simulink model "gm_sampleModel1476_sub"  (R2023a)
settings: Solver=VariableStepAuto  StartTime=0.0  StopTime=10.0  RelTol=1e-3
libraries: simulink x1
settings Model: Creator=user1  LastModifiedBy=user1
settings OptimizationCC: BlockReduction=off  ConditionallyExecuteInputs=off
settings DebuggingCC: InheritedTsInSrcMsg=none

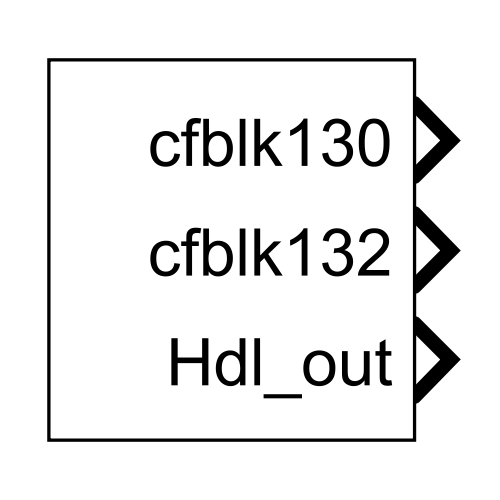
[thumbnail: Simulink's stored preview of the top-level diagram]
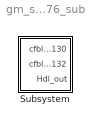
== system gm_sampleModel1476_sub ==
  Subsystem : Subsystem

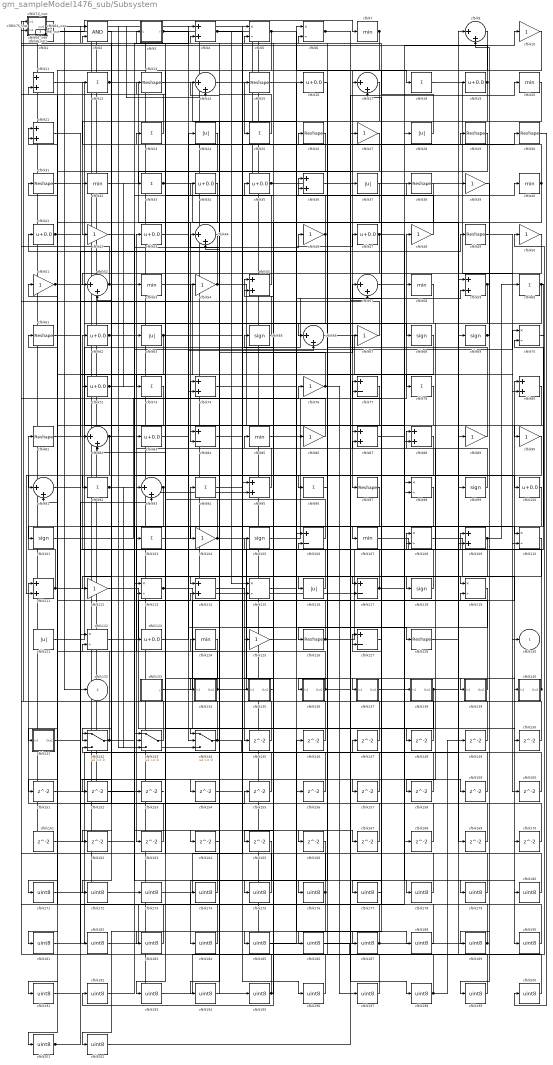
== system gm_sampleModel1476_sub/Subsystem ==
  cfblk1 : simulink/Logic and Bit Operations/Extract Bits  bitsToExtract=Upper half  numBits=8  bitIdxRange=[0 7]  outScalingMode=Preserve fixed-point scaling
      settings: LibrarySourceBlock=|
      | hdlsllib/Logic and Bit
      | Operations/Extract Bits
  cfblk{10,27,39,42,46,48,50..51,54,67,76,86,89..90,104,112,125} (17 alike) : Gain  OutDataTypeStr=uint8
  cfblk{16,19,34..35,41,43,47,62,72,83,100,123} (12 alike) : Bias  Bias=0.0  SaturateOnIntegerOverflow=off
  cfblk{65,68..69,99,101,105,118} (7 alike) : Signum
  cfblk102_inst : Subsystem
  cfblk{12,18,23,25,33,60,73,78,92,94,96,103} (12 alike) : Sum  Inputs=+  OutDataTypeStr=uint8
  cfblk{77,84,106,117,127} (5 alike) : Sum  Inputs=+-  OutDataTypeStr=uint8
  cfblk{7,20,32,40,53,58,85,107,124} (9 alike) : MinMax  OutDataTypeStr=uint8
  cfblk{5..6,70,98,108,110,113,115,119,122} (10 alike) : Product  Inputs=*/  OutDataTypeStr=uint8  RndMeth=Zero  SaturateOnIntegerOverflow=on
  cfblk{4,11,21,36,55,59,74,80,87..88,95,109,111,114} (14 alike) : Sum  OutDataTypeStr=uint8
  cfblk{24,28,37,63,116,121} (6 alike) : Abs  OutDataTypeStr=uint8  SaturateOnIntegerOverflow=off
  cfblk120_inst : Subsystem
  cfblk{13,15,26,29..31,38,49,61,81,97,126,128} (13 alike) : Reshape
  cfblk133 : Subsystem  mask(Counter Free-Running){NumBits=double(16), tsamp=double(-1)}
      mask prompts: NumBits "Simulink:masks:NumberOfBits_MP"; tsamp "Simulink:masks:SampleTime_MP"
      mask help: Simulink:masks:CounterFreeRunning_MD
  cfblk134 : Subsystem
  cfblk135 : Subsystem
  cfblk136 : Subsystem
  cfblk137 : Subsystem
  cfblk138 : Subsystem
  cfblk139 : Subsystem
  cfblk{9,14,17,44,52,57,66,82,91,93} (10 alike) : Sum  Inputs=|++  OutDataTypeStr=uint8
  cfblk140 : Subsystem
  cfblk141 : Subsystem
  cfblk142 : Switch  OutDataTypeStr=uint8  SaturateOnIntegerOverflow=off  InputSameDT=off
  cfblk143 : Switch  OutDataTypeStr=uint8  SaturateOnIntegerOverflow=off  InputSameDT=off
  cfblk144 : Switch  OutDataTypeStr=uint8  SaturateOnIntegerOverflow=off  InputSameDT=off
  cfblk{145..170} (26 alike) : Delay  SampleTime=1
  cfblk{171..202} (32 alike) : DataTypeConversion  OutDataTypeStr=uint8  SaturateOnIntegerOverflow=off  RndMeth=Floor
  cfblk2 : Logic  AllPortsSameDT=off  OutDataTypeStr=boolean
  cfblk3 : Subsystem  mask(Detect Rise Positive){vinit=double(0), InputProcessing=Elements as channels (sample based), OutDataTypeStr=uint8}
      mask prompts: vinit "Simulink:masks:InitialCondition_MP"; InputProcessing "Simulink:masks:InputProcessing_MP"; OutDataTypeStr "Simulink:masks:OutputDataType_MP"
      mask help: Simulink:masks:DetectRisePositive_MD
      mask init:
      | InputProcessing = 'Elements as channels (sample based)';
      | OutDataTypeStr = 'uint8';
      | vinit = double(0);
      mask TypeOptions InputProcessing: Simulink:masks:ColumnsAsChannelsFrameBased | Simulink:masks:ElementsAsChannelsSampleBased
      mask TypeOptions OutDataTypeStr: Simulink:masks:uint8 | Simulink:masks:boolean
      mask Display: fprintf('U > 0\n&  NOT\nU/z > 0')
  cfblk45_inst : Subsystem
  cfblk56_inst : Subsystem
  cfblk64_inst : Subsystem
  cfblk71_inst : Subsystem
  cfblk75_inst : Subsystem
  cfblk8_inst : Subsystem
  cfblk130 : Outport  OutDataTypeStr=uint8  SampleTime=1  VectorParamsAs1DForOutWhenUnconnected=off
  cfblk132 : Outport  Port=2  OutDataTypeStr=uint8  SampleTime=1  VectorParamsAs1DForOutWhenUnconnected=off
  Hdl_out : Outport  Port=3  OutDataTypeStr=uint8  SampleTime=1
  wires:
  cfblk1/1 -> cfblk7/1
  cfblk10/1 -> cfblk97/1
  cfblk100/1 -> cfblk163/1
  cfblk101/1 -> cfblk76/1
  cfblk102_inst/1(out1) -> cfblk173/1
  cfblk103/1 -> cfblk94/1
  cfblk104/1 -> cfblk82/2, cfblk119/1, cfblk137/1(In1)
  cfblk105/1 -> cfblk48/1
  cfblk106/1 -> cfblk8_inst/1(in1)
  cfblk107/1 -> cfblk70/2
  cfblk108/1 -> cfblk190/1
  cfblk109/1 -> cfblk143/2, cfblk60/1
  cfblk11/1 -> cfblk87/1
  cfblk110/1 -> cfblk114/1
  cfblk111/1 -> cfblk81/1, cfblk118/1
  cfblk112/1 -> cfblk170/1
  cfblk113/1 -> cfblk30/1, cfblk150/1
  cfblk114/1 -> cfblk145/1
  cfblk115/1 -> cfblk16/1
  cfblk116/1 -> cfblk43/1
  cfblk117/1 -> cfblk105/1, cfblk10/1
  cfblk118/1 -> cfblk62/1
  cfblk119/1 -> cfblk126/1
  cfblk12/1 -> cfblk84/2, cfblk142/2
  cfblk120_inst/1(out1) -> cfblk95/2
  cfblk121/1 -> cfblk59/2
  cfblk122/1 -> cfblk114/2
  cfblk123/1 -> cfblk24/1
  cfblk124/1 -> cfblk193/1
  cfblk125/1 -> cfblk58/1
  cfblk126/1 -> cfblk109/1, cfblk51/1
  cfblk127/1 -> cfblk187/1
  cfblk128/1 -> cfblk89/1
  cfblk13/1 -> cfblk106/1
  cfblk133/1(y) -> cfblk80/1
  cfblk134/1(Out1) -> cfblk9/1, cfblk61/1
  cfblk135/1(Out1) -> cfblk55/1
  cfblk136/1(Out1) -> cfblk93/1, cfblk119/2, cfblk20/1
  cfblk137/1(Out1) -> cfblk98/2
  cfblk138/1(Out1) -> cfblk69/1, cfblk153/1
  cfblk139/1(Out1) -> cfblk44/1
  cfblk14/1 -> cfblk25/1
  cfblk140/1(Out1) -> cfblk88/1, cfblk83/1
  cfblk141/1(Out1) -> cfblk154/1
  cfblk142/1 -> cfblk123/1, cfblk46/1, cfblk164/1, cfblk122/2
  cfblk143/1 -> cfblk72/1
  cfblk144/1 -> cfblk147/1, cfblk113/2
  cfblk145/1 -> cfblk14/1
  cfblk146/1 -> cfblk120_inst/2(in2)
  cfblk147/1 -> cfblk8_inst/2(in2)
  cfblk148/1 -> cfblk87/2
  cfblk149/1 -> cfblk11/2
  cfblk15/1 -> cfblk156/1
  cfblk150/1 -> cfblk64_inst/2(in2)
  cfblk151/1 -> cfblk59/1
  cfblk152/1 -> cfblk74/1
  cfblk153/1 -> cfblk1/1
  cfblk154/1 -> cfblk115/2
  cfblk155/1 -> cfblk142/3
  cfblk156/1 -> cfblk95/1
  cfblk157/1 -> cfblk44/2
  cfblk158/1 -> cfblk6/2
  cfblk159/1 -> cfblk2/2
  cfblk16/1 -> cfblk96/1
  cfblk160/1 -> cfblk106/2
  cfblk161/1 -> cfblk143/1
  cfblk162/1 -> cfblk70/1
  cfblk163/1 -> cfblk111/1
  cfblk164/1 -> cfblk4/2
  cfblk165/1 -> cfblk184/1
  cfblk166/1 -> cfblk192/1
  cfblk167/1 -> cfblk5/2
  cfblk168/1 -> cfblk98/1
  cfblk169/1 -> cfblk52/2
  cfblk17/1 -> cfblk104/1
  cfblk170/1 -> cfblk17/2
  cfblk171/1 -> cfblk63/1
  cfblk172/1 -> cfblk38/1
  cfblk173/1 -> cfblk15/1
  cfblk174/1 -> cfblk102_inst/1(in1)
  cfblk175/1 -> cfblk102_inst/2(in2)
  cfblk176/1 -> cfblk31/1, cfblk202/1, cfblk175/1, cfblk113/1
  cfblk177/1 -> cfblk77/1
  cfblk178/1 -> cfblk77/2
  cfblk179/1 -> cfblk13/1
  cfblk18/1 -> cfblk130/1
  cfblk180/1 -> cfblk57/1
  cfblk181/1 -> cfblk57/2
  cfblk182/1 -> cfblk28/1
  cfblk183/1 -> cfblk21/1
  cfblk184/1 -> cfblk21/2
  cfblk185/1 -> cfblk146/1
  cfblk186/1 -> cfblk50/1
  cfblk187/1 -> cfblk186/1, cfblk122/1
  cfblk188/1 -> cfblk127/1
  cfblk189/1 -> cfblk127/2, Hdl_out/1
  cfblk19/1 -> cfblk66/1, cfblk56_inst/2(in2)
  cfblk190/1 -> cfblk64_inst/1(in1)
  cfblk191/1 -> cfblk108/1
  cfblk192/1 -> cfblk108/2
  cfblk193/1 -> cfblk19/1
  cfblk194/1 -> cfblk124/1
  cfblk195/1 -> cfblk56_inst/1(in1), cfblk85/1
  cfblk196/1 -> cfblk75_inst/1(in1)
  cfblk197/1 -> cfblk75_inst/2(in2)
  cfblk198/1 -> cfblk35/1, cfblk149/1
  cfblk199/1 -> cfblk36/1
  cfblk2/1 -> cfblk172/1
  cfblk20/1 -> cfblk42/1
  cfblk200/1 -> cfblk36/2
  cfblk201/1 -> cfblk93/2, cfblk174/1, cfblk155/1
  cfblk202/1 -> cfblk27/1
  cfblk21/1 -> cfblk182/1
  cfblk23/1 -> cfblk45_inst/1(in1)
  cfblk24/1 -> cfblk91/1
  cfblk25/1 -> cfblk2/1
  cfblk26/1 -> cfblk134/1(In1)
  cfblk27/1 -> cfblk201/1
  cfblk28/1 -> cfblk120_inst/1(in1)
  cfblk29/1 -> cfblk32/1
  cfblk3/1(Y) -> cfblk66/2, cfblk128/1
  cfblk30/1 -> cfblk200/1
  cfblk31/1 -> cfblk157/1
  cfblk32/1 -> cfblk37/1
  cfblk33/1 -> cfblk99/1, cfblk169/1
  cfblk34/1 -> cfblk103/1
  cfblk35/1 -> cfblk188/1, cfblk148/1
  cfblk36/1 -> cfblk198/1
  cfblk37/1 -> cfblk73/1
  cfblk38/1 -> cfblk171/1
  cfblk39/1 -> cfblk199/1
  cfblk4/1 -> cfblk166/1, cfblk115/1
  cfblk40/1 -> cfblk165/1, cfblk135/1(In1), cfblk12/1
  cfblk41/1 -> cfblk82/1, cfblk78/1
  cfblk42/1 -> cfblk100/1
  cfblk43/1 -> cfblk140/1(In1)
  cfblk44/1 -> cfblk142/1
  cfblk45_inst/1(out1) -> cfblk121/1
  cfblk46/1 -> cfblk144/1, cfblk6/1
  cfblk47/1 -> cfblk88/2, cfblk112/1
  cfblk48/1 -> cfblk26/1
  cfblk49/1 -> cfblk80/2
  cfblk5/1 -> cfblk183/1, cfblk18/1
  cfblk50/1 -> cfblk185/1
  cfblk51/1 -> cfblk144/2, cfblk138/1(In1)
  cfblk52/1 -> cfblk45_inst/2(in2), cfblk33/1
  cfblk53/1 -> cfblk86/1
  cfblk54/1 -> cfblk52/1, cfblk168/1
  cfblk55/1 -> cfblk23/1
  cfblk56_inst/1(out1) -> cfblk161/1
  cfblk57/1 -> cfblk179/1
  cfblk58/1 -> cfblk92/1
  cfblk59/1 -> cfblk74/2, cfblk189/1
  cfblk6/1 -> cfblk68/1, cfblk109/2
  cfblk60/1 -> cfblk158/1, cfblk110/1
  cfblk61/1 -> cfblk49/1
  cfblk62/1 -> cfblk84/1, cfblk4/1, cfblk167/1
  cfblk63/1 -> cfblk101/1, cfblk5/1
  cfblk64_inst/1(out1) -> cfblk144/3, cfblk11/1
  cfblk65/1 -> cfblk55/2
  cfblk66/1 -> cfblk160/1
  cfblk67/1 -> cfblk71_inst/2(in2)
  cfblk68/1 -> cfblk136/1(In1)
  cfblk69/1 -> cfblk9/2, cfblk29/1
  cfblk7/1 -> cfblk181/1, cfblk17/1
  cfblk70/1 -> cfblk90/1
  cfblk71_inst/1(out1) -> cfblk117/2, cfblk39/1
  cfblk72/1 -> cfblk159/1, cfblk53/1
  cfblk73/1 -> cfblk141/1(In1)
  cfblk74/1 -> cfblk139/1(In1)
  cfblk75_inst/1(out1) -> cfblk195/1
  cfblk76/1 -> cfblk34/1, cfblk197/1
  cfblk77/1 -> cfblk176/1
  cfblk78/1 -> cfblk91/2
  cfblk8_inst/1(out1) -> cfblk14/2, cfblk132/1
  cfblk80/1 -> cfblk194/1
  cfblk81/1 -> cfblk54/1
  cfblk82/1 -> cfblk117/1, cfblk111/2
  cfblk83/1 -> cfblk40/1
  cfblk84/1 -> cfblk67/1
  cfblk85/1 -> cfblk47/1
  cfblk86/1 -> cfblk71_inst/1(in1)
  cfblk87/1 -> cfblk180/1
  cfblk88/1 -> cfblk125/1
  cfblk89/1 -> cfblk41/1
  cfblk9/1 -> cfblk177/1
  cfblk90/1 -> cfblk191/1
  cfblk91/1 -> cfblk110/2
  cfblk92/1 -> cfblk178/1, cfblk143/3
  cfblk93/1 -> cfblk152/1, cfblk151/1
  cfblk94/1 -> cfblk196/1
  cfblk95/1 -> cfblk3/1(U)
  cfblk96/1 -> cfblk116/1
  cfblk97/1 -> cfblk162/1
  cfblk98/1 -> cfblk107/1
  cfblk99/1 -> cfblk65/1

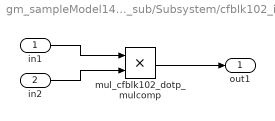
== system gm_sampleModel1476_sub/Subsystem/cfblk102_inst ==
  in1 : Inport  OutDataTypeStr=uint8  SampleTime=1
  in2 : Inport  Port=2  OutDataTypeStr=uint8  SampleTime=1
  mul_cfblk102_dotp_mulcomp : Product  Inputs=**  OutDataTypeStr=uint8  SampleTime=1
  out1 : Outport  OutDataTypeStr=uint8  SampleTime=1
  wires:
  in1/1 -> mul_cfblk102_dotp_mulcomp/1
  in2/1 -> mul_cfblk102_dotp_mulcomp/2
  mul_cfblk102_dotp_mulcomp/1 -> out1/1

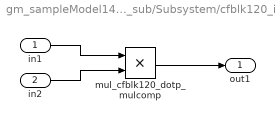
== system gm_sampleModel1476_sub/Subsystem/cfblk120_inst ==
  in1 : Inport  OutDataTypeStr=uint8  SampleTime=1
  in2 : Inport  Port=2  OutDataTypeStr=uint8  SampleTime=1
  mul_cfblk120_dotp_mulcomp : Product  Inputs=**  OutDataTypeStr=uint8  SampleTime=1
  out1 : Outport  OutDataTypeStr=uint8  SampleTime=1
  wires:
  in1/1 -> mul_cfblk120_dotp_mulcomp/1
  in2/1 -> mul_cfblk120_dotp_mulcomp/2
  mul_cfblk120_dotp_mulcomp/1 -> out1/1

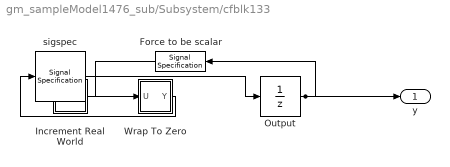
== system gm_sampleModel1476_sub/Subsystem/cfblk133 ==
  Force to be scalar : SignalSpecification  DisableCoverage=on  Dimensions=1
  Increment Real World : Subsystem  mask(Real World Value Increment){}
      mask help: Simulink:masks:RealWorldValueIncrement_MD
      mask Display: disp('V++')
  Output : UnitDelay  InitialCondition=0.0  SampleTime=tsamp  HasFrameUpgradeWarning=on
  Wrap To Zero : Subsystem  mask(Wrap To Zero){Threshold=double(65535)}
      mask prompts: Threshold "Simulink:masks:Threshold_MP"
      mask help: Simulink:masks:WrapToZero_MD
  sigspec : SignalSpecification  OutDataTypeStr=uint16  Dimensions=1
  y : Outport  SampleTime=1
  wires:
  Force to be scalar/1 -> Increment Real World/1(u)
  Increment Real World/1(y) -> Wrap To Zero/1(U)
  Output/1 -> Force to be scalar/1, y/1
  Wrap To Zero/1(Y) -> sigspec/1
  sigspec/1 -> Output/1

== system gm_sampleModel1476_sub/Subsystem/cfblk134 ==
  In1 : Inport  OutDataTypeStr=uint8  PortDimensions=1  SampleTime=1
  Out1 : Outport  SampleTime=1
  wires:
  In1/1 -> Out1/1

== system gm_sampleModel1476_sub/Subsystem/cfblk135 ==
  In1 : Inport  OutDataTypeStr=uint8  PortDimensions=1  SampleTime=1
  Out1 : Outport  SampleTime=1
  wires:
  In1/1 -> Out1/1

== system gm_sampleModel1476_sub/Subsystem/cfblk136 ==
  In1 : Inport  OutDataTypeStr=uint8  PortDimensions=1  SampleTime=1
  Out1 : Outport  SampleTime=1
  wires:
  In1/1 -> Out1/1

== system gm_sampleModel1476_sub/Subsystem/cfblk137 ==
  In1 : Inport  OutDataTypeStr=uint8  PortDimensions=1  SampleTime=1
  Out1 : Outport  SampleTime=1
  wires:
  In1/1 -> Out1/1

== system gm_sampleModel1476_sub/Subsystem/cfblk138 ==
  In1 : Inport  OutDataTypeStr=uint8  PortDimensions=1  SampleTime=1
  Out1 : Outport  SampleTime=1
  wires:
  In1/1 -> Out1/1

== system gm_sampleModel1476_sub/Subsystem/cfblk139 ==
  In1 : Inport  OutDataTypeStr=uint8  PortDimensions=1  SampleTime=1
  Out1 : Outport  SampleTime=1
  wires:
  In1/1 -> Out1/1

== system gm_sampleModel1476_sub/Subsystem/cfblk140 ==
  In1 : Inport  OutDataTypeStr=uint8  PortDimensions=1  SampleTime=1
  Out1 : Outport  SampleTime=1
  wires:
  In1/1 -> Out1/1

== system gm_sampleModel1476_sub/Subsystem/cfblk141 ==
  In1 : Inport  OutDataTypeStr=uint8  PortDimensions=1  SampleTime=1
  Out1 : Outport  SampleTime=1
  wires:
  In1/1 -> Out1/1

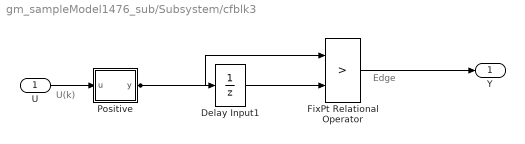
== system gm_sampleModel1476_sub/Subsystem/cfblk3 ==
  note: U(k)
  note: Edge
  U : Inport  OutDataTypeStr=uint8  SampleTime=1
  Delay Input1 : UnitDelay  Description=Store in Global RAM  DisableCoverage=on  InitialCondition=vinit  SampleTime=-1  HasFrameUpgradeWarning=on
  FixPt Relational Operator : RelationalOperator  Operator=>  OutDataTypeStr=fixdt(0, 8)  ZeroCross=off  InputSameDT=off
  Positive : Subsystem  mask(Compare To Zero){relop=>, OutDataTypeStr=boolean, ZeroCross=off}
      mask prompts: relop "Simulink:masks:Operator_MP"; OutDataTypeStr "Simulink:masks:OutputDataType_MP"; ZeroCross "Simulink:masks:EnableZerocrossingDetection_MP"
      mask help: Simulink:masks:CompareToZero_MD
      mask init:
      | OutDataTypeStr = 'boolean';
      | ZeroCross = 'off';
      | blkName = 'sampleModel1476_sub/Subsystem/cfblk3/Positive';
      | relop = '>';
      | setValue = 'boolean';
      mask TypeOptions relop: == | ~= | < | <= | >= | >
      mask TypeOptions OutDataTypeStr: Simulink:masks:uint8 | Simulink:masks:boolean
      mask Callback ZeroCross: sl('zeroCrossEnable', gcbh);
      mask Display: disp([relop,' 0'])
  Y : Outport  SampleTime=1
  wires:
  U/1 -> Positive/1(u)
  Delay Input1/1 -> FixPt Relational Operator/2
  FixPt Relational Operator/1 -> Y/1
  Positive/1(y) -> FixPt Relational Operator/1, Delay Input1/1

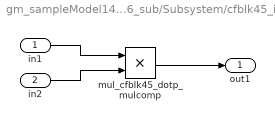
== system gm_sampleModel1476_sub/Subsystem/cfblk45_inst ==
  in1 : Inport  OutDataTypeStr=uint8  SampleTime=1
  in2 : Inport  Port=2  OutDataTypeStr=uint8  SampleTime=1
  mul_cfblk45_dotp_mulcomp : Product  Inputs=**  OutDataTypeStr=uint8  SampleTime=1
  out1 : Outport  OutDataTypeStr=uint8  SampleTime=1
  wires:
  in1/1 -> mul_cfblk45_dotp_mulcomp/1
  in2/1 -> mul_cfblk45_dotp_mulcomp/2
  mul_cfblk45_dotp_mulcomp/1 -> out1/1

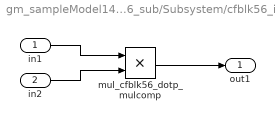
== system gm_sampleModel1476_sub/Subsystem/cfblk56_inst ==
  in1 : Inport  OutDataTypeStr=uint8  SampleTime=1
  in2 : Inport  Port=2  OutDataTypeStr=uint8  SampleTime=1
  mul_cfblk56_dotp_mulcomp : Product  Inputs=**  OutDataTypeStr=uint8  SampleTime=1
  out1 : Outport  OutDataTypeStr=uint8  SampleTime=1
  wires:
  in1/1 -> mul_cfblk56_dotp_mulcomp/1
  in2/1 -> mul_cfblk56_dotp_mulcomp/2
  mul_cfblk56_dotp_mulcomp/1 -> out1/1

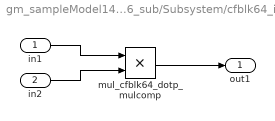
== system gm_sampleModel1476_sub/Subsystem/cfblk64_inst ==
  in1 : Inport  OutDataTypeStr=uint8  SampleTime=1
  in2 : Inport  Port=2  OutDataTypeStr=uint8  SampleTime=1
  mul_cfblk64_dotp_mulcomp : Product  Inputs=**  OutDataTypeStr=uint8  SampleTime=1
  out1 : Outport  OutDataTypeStr=uint8  SampleTime=1
  wires:
  in1/1 -> mul_cfblk64_dotp_mulcomp/1
  in2/1 -> mul_cfblk64_dotp_mulcomp/2
  mul_cfblk64_dotp_mulcomp/1 -> out1/1

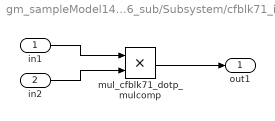
== system gm_sampleModel1476_sub/Subsystem/cfblk71_inst ==
  in1 : Inport  OutDataTypeStr=uint8  SampleTime=1
  in2 : Inport  Port=2  OutDataTypeStr=uint8  SampleTime=1
  mul_cfblk71_dotp_mulcomp : Product  Inputs=**  OutDataTypeStr=uint8  SampleTime=1
  out1 : Outport  OutDataTypeStr=uint8  SampleTime=1
  wires:
  in1/1 -> mul_cfblk71_dotp_mulcomp/1
  in2/1 -> mul_cfblk71_dotp_mulcomp/2
  mul_cfblk71_dotp_mulcomp/1 -> out1/1

== system gm_sampleModel1476_sub/Subsystem/cfblk75_inst ==
  in1 : Inport  OutDataTypeStr=uint8  SampleTime=1
  in2 : Inport  Port=2  OutDataTypeStr=uint8  SampleTime=1
  mul_cfblk75_dotp_mulcomp : Product  Inputs=**  OutDataTypeStr=uint8  SampleTime=1
  out1 : Outport  OutDataTypeStr=uint8  SampleTime=1
  wires:
  in1/1 -> mul_cfblk75_dotp_mulcomp/1
  in2/1 -> mul_cfblk75_dotp_mulcomp/2
  mul_cfblk75_dotp_mulcomp/1 -> out1/1

== system gm_sampleModel1476_sub/Subsystem/cfblk8_inst ==
  in1 : Inport  OutDataTypeStr=uint8  SampleTime=1
  in2 : Inport  Port=2  OutDataTypeStr=uint8  SampleTime=1
  mul_cfblk8_dotp_mulcomp : Product  Inputs=**  OutDataTypeStr=uint8  SampleTime=1
  out1 : Outport  OutDataTypeStr=uint8  SampleTime=1
  wires:
  in1/1 -> mul_cfblk8_dotp_mulcomp/1
  in2/1 -> mul_cfblk8_dotp_mulcomp/2
  mul_cfblk8_dotp_mulcomp/1 -> out1/1

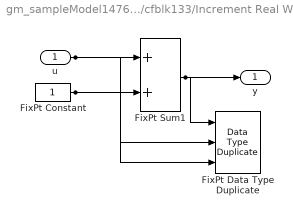
== system gm_sampleModel1476_sub/Subsystem/cfblk133/Increment Real World ==
  u : Inport  OutDataTypeStr=uint16  SampleTime=1
  FixPt Constant : Constant  DisableCoverage=on  OutDataTypeStr=Inherit: Inherit via back propagation  SampleTime=-1
  FixPt Data Type Duplicate : DataTypeDuplicate  DisableCoverage=on  NumInputPorts=3
  FixPt Sum1 : Sum  InputSameDT=on  OutDataTypeStr=Inherit: Inherit via back propagation  LockScale=on
  y : Outport  SampleTime=1
  wires:
  u/1 -> FixPt Sum1/1, FixPt Data Type Duplicate/2
  FixPt Constant/1 -> FixPt Sum1/2, FixPt Data Type Duplicate/3
  FixPt Sum1/1 -> FixPt Data Type Duplicate/1, y/1

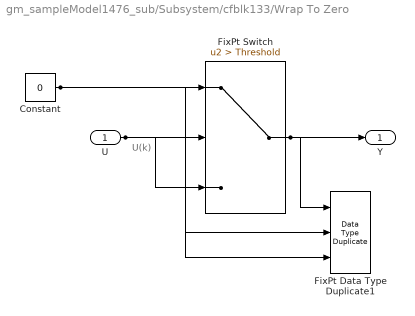
== system gm_sampleModel1476_sub/Subsystem/cfblk133/Wrap To Zero ==
  note: U(k)
  U : Inport  OutDataTypeStr=uint16  SampleTime=1
  Constant : Constant  DisableCoverage=on  Value=0  OutDataTypeStr=Inherit: Inherit via back propagation  SampleTime=-1
  FixPt Data Type Duplicate1 : DataTypeDuplicate  DisableCoverage=on  NumInputPorts=3
  FixPt Switch : Switch  Criteria=u2 > Threshold  Threshold=Threshold  OutDataTypeStr=Inherit: Inherit via back propagation  ZeroCross=off  SaturateOnIntegerOverflow=off  InputSameDT=off
  Y : Outport  SampleTime=1
  wires:
  U/1 -> FixPt Switch/3, FixPt Switch/2, FixPt Data Type Duplicate1/2
  Constant/1 -> FixPt Switch/1, FixPt Data Type Duplicate1/3
  FixPt Switch/1 -> FixPt Data Type Duplicate1/1, Y/1

== system gm_sampleModel1476_sub/Subsystem/cfblk3/Positive ==
  u : Inport  OutDataTypeStr=uint8  SampleTime=1
  Compare : RelationalOperator  Operator=>  OutDataTypeStr=boolean  ZeroCross=off
  Constant : Constant  DisableCoverage=on  Value=0  OutDataTypeStr=Inherit: Inherit via back propagation  SampleTime=-1  PreserveConstantTs=on
  y : Outport  SampleTime=1
  wires:
  u/1 -> Compare/1
  Compare/1 -> y/1
  Constant/1 -> Compare/2
